simulink model "hyd_hyb_2_int_cont_Final_AMT"  (R2013b)
settings: Solver=ode4  StartTime=0  StopTime=3005  FixedStep=0.01  MaxStep=.4  RelTol=1e-8
InitFcn:
  | const_3_new
values from neighbouring files (symbols this model uses):
  Af = 6.3    [brk_enrg.m]    (also in brk_enrg_1.m)
  BSFC_906_205 = [3.5684 4.3466 5.1668 6.0769 6.988 7.8992 8.8104 9.7336 10.8548 11.9809 13.1112 14.2571 ... (663 elements, 39x17)]    [BSFC_map_906_205.mat]
  Cd = 0.55    [brk_enrg.m]    (also in brk_enrg_1.m)
  den = 1.202    [brk_enrg.m]    (also in brk_enrg_1.m)
  fr = 0.01    [brk_enrg.m]    (also in brk_enrg_1.m)
undefined symbols (not defined in the file or in its folder): clutchRise, down_spd_2, down_spd_3, down_spd_4, down_spd_c, Driving_Cycle, fuel_density, gearshift, I_wheel, Idle_spd_eng_906, M1_hydr, p_v_15, pmax_125, qv_125, Rw, sec_eng_sfc_map, T0, T1, T_max_906, T_min, TC_spd_ratio_max, teta_new_10, torque_convertor, Twait, up_spd_1, up_spd_2, up_spd_3, up_spd_c, v_p_10, v_p_15, v_p_5
libraries: neural x1742, fl_lib x43, nesl_utility x30, sdl_lib x14, simulink x4, simulink_need_slupdate x1
(part 11 of 26)

== system hyd_hyb_2_int_cont_Final_AMT/controller1/optimized controller/SOC upper 0.5/SOC under 0.6/net_col_e_f_5_6/Layer 2/LW{2,1} ==
  "ad{2,1}" : Inport  PortDimensions=30
  "IW{2,1}(1,:)'" : Constant  Value=[-0.030393832532962472;-0.2140586465492049;-0.31177410134924299;-0.46613714335472767;-0.201873752791425;-0.35802654413849078;0.41211751545428793;-0.35557829317260753;0.17263895513984945;-0.21666908912043678;-0.13972381535234679;-0.019824875407318664;0.17842229946428553;0.044381204849071522;-0.32894732465246224;-0.12171008049632184;0.13814590271554272;0.31343496753063571;0.49075574510674602;-0.07753439785263945;-0.11371475039833147;-0.43264143413308215;-0.31682924708133714;0.45184843514620843;-0.10010733916402992;-0.073217200056284279;0.33498722182306373;0.2080296291338882;-0.34019436744511455;-0.12407925676720709]
  "IW{2,1}(10,:)'" : Constant  Value=[-0.2505704282524524;-0.3939257554207935;-0.29975165870681642;-0.15031973290133904;-0.24045771892346329;-0.24216831733474872;0.34991520385977254;0.056483630435657121;0.075039420272193916;0.040783928391016355;-0.17972854864617466;0.37100873007899093;0.3223440043286851;0.083094181567428288;-0.34343211957443465;-0.24139719218091207;-0.23310945944076636;-0.19630209941555543;-0.39839647141125911;-0.086263558874944163;0.084290908148239183;0.46372794004131584;0.30745835414815731;0.4667718683031023;0.38177352303007822;0.39526221301583331;0.037058129894969059;-0.033237412446624953;0.085864544510327004;-0.4416572811793027]
  "IW{2,1}(2,:)'" : Constant  Value=[-0.28762870212077329;0.054589128164715936;0.43070941004987917;-0.19143207832331097;0.0318475712201398;-0.053702387359868146;0.3782037039878825;-0.10929522120960172;0.02340575506249706;0.1208551424159988;-0.32907776200005534;-0.29614820983664508;-0.04883438578651441;0.2945504283388431;0.38772134611455616;-0.1426067233264004;0.34279273527863979;-0.42587520602132178;0.30745629555523329;0.085481158280511255;-0.31301428028501527;0.45433653176700362;-0.34548226823741135;0.45162137833646937;-0.19606462470782865;-0.44727339366708768;-0.32633196267115394;-0.022768106510234126;0.19019249866074842;0.12534221654070224]
  "IW{2,1}(3,:)'" : Constant  Value=[0.39112741680931812;-0.31978339521640231;-0.45618332838328646;0.22187613151776697;0.15902090508890185;0.083633472465386507;0.068775436612897214;-0.27468778024818002;-0.0095156153879017956;-0.3329705145032763;-0.41709465282714198;-0.083926949400729201;-0.43867924463374353;-0.47594030290625516;0.37055116856733306;-0.30038080956129914;-0.19346252510558046;-0.071156466707070598;-0.1565410346606585;0.31532679870256697;-0.25473325292829679;0.33712413893538379;-0.085088376218202588;-0.17938172910409972;0.24970446460562623;-0.33450621725925617;-0.17977936758544141;0.30664510288542302;-0.068953816926079908;-0.13239439222807625]
  "IW{2,1}(4,:)'" : Constant  Value=[0.5236702898730865;0.21199966696477551;0.35952752928707649;0.019723530590060441;0.44209036013212977;-0.045784888845008344;0.54989711619444792;-0.047025448166544644;-0.036356167286904967;0.24149337951075159;-0.36033388484015128;0.15509905661754866;0.24429431465823442;0.56993242132756905;-0.046193773380533189;-0.16184817194805917;0.17925337861437229;0.46969723879260278;0.34350789605630055;0.08863875089456541;0.20464674967063287;0.21542542386226093;-0.30757414976248237;0.22245003609036712;0.099301281549722578;0.04057872191728587;-0.33201719417637826;-0.47694799309855712;-0.33359512873481728;-0.33443453741741941]
  "IW{2,1}(5,:)'" : Constant  Value=[-0.39959821967519593;-0.31362810096707033;-0.31682724713016341;0.39862604414021602;-0.36168966900035454;-0.38588696726317745;-0.15797698948252611;-0.090531432147917826;-0.33017756180156344;-0.36582779220206285;-0.16339659393293465;0.30719233431666931;-0.37016484251633996;0.344361440321791;-0.17456285655515369;0.2131417301444393;-0.32163373894503566;-0.29509333147520467;0.14907288465152124;-0.31687539569313966;0.11409578709933664;0.16969225538936128;-0.1613998950013931;0.11147161080246354;0.11126677588053642;-0.10582537476789625;0.37764324773258484;-0.25725888409799397;0.17346828146213097;0.2968195483551983]
  "IW{2,1}(6,:)'" : Constant  Value=[-0.11716752768262495;0.20377807736649567;0.39051919150098868;-0.10068145034167778;-0.45898166603392643;0.14044780715231203;0.3766843442574494;-0.31621402495343004;0.40628439400051353;0.0026886561759890833;-0.23275447184164255;0.11741623482208553;-0.47709346258154012;0.029795882252597751;0.27610056922766701;0.11975856223889453;-0.23493711394866479;0.39441111981074417;-0.1305257437571978;-0.3096269494893204;0.21423914366738864;0.29007697061490489;-0.37128870036285971;-0.17096385603206457;-0.33949208301054939;-0.20358861932336775;-0.103794175225949;-0.12728191492578217;0.073028592828514385;0.50715491081104047]
  "IW{2,1}(7,:)'" : Constant  Value=[0.22889715197947469;-0.14817850016315076;0.29384797220436742;-0.17292464780674385;0.039905368244081973;0.51560989905964549;-0.019104485775315299;0.00450671459486187;-0.24885944976112842;0.11294055983311714;-0.35984134998870648;0.56660710621235377;0.4502529330165625;-0.12729977158914091;-0.25887898451001889;-0.4202593621623692;0.079298806675420247;0.23489367335784675;-0.36990629226240712;0.049141324657233795;0.16139682719459081;-0.30821522108094518;0.13499998583520637;-0.089586453672634944;0.38220329351721338;-0.26661160481608931;-0.14550662761818581;-0.13187580715835978;-0.11647199599773699;0.26317272202300696]
  "IW{2,1}(8,:)'" : Constant  Value=[0.044685744582128734;-0.1908844366489017;-0.174794908065215;0.32643162068799214;-0.37050611537088302;-0.32225071082540269;-0.29490940136720639;0.05038227814640945;-0.42624323738224995;0.39773459662235627;-0.30823260303902394;0.18941270558875947;0.076728852910635137;-0.24291076735984238;0.040687603382098023;0.38406554522818398;-0.12119441015776648;0.54700185417442515;0.092888736216969123;0.015603285313999743;-0.4911935537467782;-0.024179836928880958;-0.14313432950027993;-0.14638852747492093;0.40459554299034611;-0.37124396054958153;0.4052460971208755;-0.1241390298447143;0.22476477752652688;0.17000260780043774]
  "IW{2,1}(9,:)'" : Constant  Value=[0.40187325571425492;0.25449281632989129;-0.076943631829698544;-0.21240760751343882;0.040048997970771043;0.19620197480948465;-0.37138567337556944;0.39831762613048866;-0.28931266215843032;-0.39729083923611486;-0.46921791995515649;0.51412890115003618;0.31379829123446729;0.095315428974239447;-0.44370143634003684;-0.33140964460964284;-0.27278751479859847;-0.42011098303670114;-0.024084561465198988;0.10358437043932962;0.64313064936086206;-0.081503436078471866;-0.11002880065828506;-0.23916583284587656;0.23096285494640126;-0.19893311012086728;0.28091952945331422;-0.046984031602095543;0.24418233822697555;0.24118329610468914]
  Mux : Mux  Inputs=10
  dotprod{1..10} (10 alike) : neural/Weight Functions/dotprod
  "lz{2,1}" : Outport
  wires:
  "IW{2,1}(1,:)'"/1 -> dotprod1/1
  "ad{2,1}"/1 -> dotprod1/2, dotprod2/2, dotprod3/2, dotprod4/2, dotprod5/2, dotprod6/2, dotprod7/2, dotprod8/2, dotprod9/2, dotprod10/2
  dotprod1/1 -> Mux/1
  "IW{2,1}(2,:)'"/1 -> dotprod2/1
  dotprod2/1 -> Mux/2
  "IW{2,1}(3,:)'"/1 -> dotprod3/1
  dotprod3/1 -> Mux/3
  "IW{2,1}(4,:)'"/1 -> dotprod4/1
  dotprod4/1 -> Mux/4
  "IW{2,1}(5,:)'"/1 -> dotprod5/1
  dotprod5/1 -> Mux/5
  "IW{2,1}(6,:)'"/1 -> dotprod6/1
  dotprod6/1 -> Mux/6
  "IW{2,1}(7,:)'"/1 -> dotprod7/1
  dotprod7/1 -> Mux/7
  "IW{2,1}(8,:)'"/1 -> dotprod8/1
  dotprod8/1 -> Mux/8
  "IW{2,1}(9,:)'"/1 -> dotprod9/1
  dotprod9/1 -> Mux/9
  "IW{2,1}(10,:)'"/1 -> dotprod10/1
  dotprod10/1 -> Mux/10
  Mux/1 -> "lz{2,1}"/1

== system hyd_hyb_2_int_cont_Final_AMT/controller1/optimized controller/SOC upper 0.5/SOC under 0.6/net_col_e_f_5_6/Layer 3/Delays 1 ==
  "p{3}" : Inport  PortDimensions=10
  mux : Mux  Inputs=1
  "pd{3,2}" : Outport
  wires:
  "p{3}"/1 -> mux/1
  mux/1 -> "pd{3,2}"/1

== system hyd_hyb_2_int_cont_Final_AMT/controller1/optimized controller/SOC upper 0.5/SOC under 0.6/net_col_e_f_5_6/Layer 3/LW{3,2} ==
  "ad{3,2}" : Inport  PortDimensions=10
  "IW{3,2}(1,:)'" : Constant  Value=[0.6820311486021321;-0.48687596019537038;-0.099773750784149948;0.92745064423738854;0.58814782146156741;-0.41412122914754468;-0.27711602366879279;0.34179434137314957;-0.92605251129828714;1.0113598211442618]
  Mux : Mux  Inputs=1
  dotprod1 : neural/Weight Functions/dotprod
  "lz{3,2}" : Outport
  wires:
  "IW{3,2}(1,:)'"/1 -> dotprod1/1
  "ad{3,2}"/1 -> dotprod1/2
  dotprod1/1 -> Mux/1
  Mux/1 -> "lz{3,2}"/1

== system hyd_hyb_2_int_cont_Final_AMT/controller1/optimized controller/SOC upper 0.5/SOC under 0.6/net_loc_rod_5_6/Layer 1/Delays 1 ==
  "p{1}" : Inport  PortDimensions=2
  mux : Mux  Inputs=1
  "pd{1,1}" : Outport
  wires:
  "p{1}"/1 -> mux/1
  mux/1 -> "pd{1,1}"/1

== system hyd_hyb_2_int_cont_Final_AMT/controller1/optimized controller/SOC upper 0.5/SOC under 0.6/net_loc_rod_5_6/Layer 1/IW{1,1} ==
  "pd{1,1}" : Inport  PortDimensions=2
  "IW{1,1}(1,:)'" : Constant  Value=[-6.7309330170199999;5.7367344667021127]
  "IW{1,1}(10,:)'" : Constant  Value=[-8.7922870682239527;1.0330077469568615]
  "IW{1,1}(11,:)'" : Constant  Value=[6.9837130293121303;5.4192670047826033]
  "IW{1,1}(12,:)'" : Constant  Value=[4.325460244122568;7.7438798911268565]
  "IW{1,1}(13,:)'" : Constant  Value=[-6.3344127461650013;6.1856486901229077]
  "IW{1,1}(14,:)'" : Constant  Value=[-1.9733514180291731;-8.6238469824021387]
  "IW{1,1}(15,:)'" : Constant  Value=[-2.3605885459119227;-8.5314691020515863]
  "IW{1,1}(16,:)'" : Constant  Value=[-4.8892080793798369;7.3866903131456692]
  "IW{1,1}(17,:)'" : Constant  Value=[5.8569397262097889;6.7096509511682889]
  "IW{1,1}(18,:)'" : Constant  Value=[-4.4027205889575827;7.6822038939167063]
  "IW{1,1}(19,:)'" : Constant  Value=[8.7792518860140909;1.1591702425203565]
  "IW{1,1}(2,:)'" : Constant  Value=[6.2678488323062229;6.251648838835326]
  "IW{1,1}(20,:)'" : Constant  Value=[-7.9610155557707865;-3.8802632991194277]
  "IW{1,1}(21,:)'" : Constant  Value=[5.755058346987636;6.7197585570713629]
  "IW{1,1}(22,:)'" : Constant  Value=[7.3858749888249431;-4.8854449488948442]
  "IW{1,1}(23,:)'" : Constant  Value=[-2.5028469102563147;-8.4893261832660354]
  "IW{1,1}(24,:)'" : Constant  Value=[8.50910667173771;-2.4597062713706324]
  "IW{1,1}(25,:)'" : Constant  Value=[-8.2476309100150864;3.2111046237292071]
  "IW{1,1}(26,:)'" : Constant  Value=[-4.0253091511868995;-7.862701807156669]
  "IW{1,1}(27,:)'" : Constant  Value=[2.2947605364640964;8.551294247952935]
  "IW{1,1}(28,:)'" : Constant  Value=[0.90305404500173392;-8.8024864439756705]
  "IW{1,1}(29,:)'" : Constant  Value=[7.0857227926174824;-5.297360563446083]
  "IW{1,1}(3,:)'" : Constant  Value=[8.4767942670534939;2.5639295625443186]
  "IW{1,1}(30,:)'" : Constant  Value=[-5.6140927717680311;-6.8589023719873676]
  "IW{1,1}(31,:)'" : Constant  Value=[-5.8556189515114712;6.6477437525997107]
  "IW{1,1}(32,:)'" : Constant  Value=[1.520259467845865;8.7265416088585415]
  "IW{1,1}(33,:)'" : Constant  Value=[-7.4255785682577606;-4.8121870145571606]
  "IW{1,1}(34,:)'" : Constant  Value=[3.7334199192712054;-7.9252934165752285]
  "IW{1,1}(35,:)'" : Constant  Value=[-8.8434135803568381;0.098556138484456934]
  "IW{1,1}(36,:)'" : Constant  Value=[8.7558988672878311;-1.1835294834309311]
  "IW{1,1}(37,:)'" : Constant  Value=[-6.3607928740217332;6.2831314432408085]
  "IW{1,1}(38,:)'" : Constant  Value=[-2.1369631047449062;-8.5869236354604546]
  "IW{1,1}(39,:)'" : Constant  Value=[-3.7481499623866923;8.0515766767633732]
  "IW{1,1}(4,:)'" : Constant  Value=[5.9639192573581292;-6.5449514183387238]
  "IW{1,1}(40,:)'" : Constant  Value=[-8.8210912896683222;1.1388181613834201]
  "IW{1,1}(5,:)'" : Constant  Value=[6.0684708526836246;6.4470542210774306]
  "IW{1,1}(6,:)'" : Constant  Value=[0.14739906835272285;8.8139730930743863]
  "IW{1,1}(7,:)'" : Constant  Value=[-4.8674516940697989;7.4037526818854085]
  "IW{1,1}(8,:)'" : Constant  Value=[5.18948242438666;-7.1849747561483799]
  "IW{1,1}(9,:)'" : Constant  Value=[-6.3190502504535511;-6.2049133477751708]
  Mux : Mux  Inputs=40
  dotprod{1..40} (40 alike) : neural/Weight Functions/dotprod
  "iz{1,1}" : Outport
  wires:
  "IW{1,1}(1,:)'"/1 -> dotprod1/1
  "pd{1,1}"/1 -> dotprod1/2, dotprod2/2, dotprod3/2, dotprod4/2, dotprod5/2, dotprod6/2, dotprod7/2, dotprod8/2, dotprod9/2, dotprod10/2, dotprod11/2, dotprod12/2, dotprod13/2, dotprod14/2, dotprod15/2, dotprod16/2, dotprod17/2, dotprod18/2, dotprod19/2, dotprod20/2, dotprod21/2, dotprod22/2, dotprod23/2, dotprod24/2, dotprod25/2, dotprod26/2, dotprod27/2, dotprod28/2, dotprod29/2, dotprod30/2, dotprod31/2, dotprod32/2, dotprod33/2, dotprod34/2, dotprod35/2, dotprod36/2, dotprod37/2, dotprod38/2, dotprod39/2, dotprod40/2
  dotprod1/1 -> Mux/1
  "IW{1,1}(2,:)'"/1 -> dotprod2/1
  dotprod2/1 -> Mux/2
  "IW{1,1}(3,:)'"/1 -> dotprod3/1
  dotprod3/1 -> Mux/3
  "IW{1,1}(4,:)'"/1 -> dotprod4/1
  dotprod4/1 -> Mux/4
  "IW{1,1}(5,:)'"/1 -> dotprod5/1
  dotprod5/1 -> Mux/5
  "IW{1,1}(6,:)'"/1 -> dotprod6/1
  dotprod6/1 -> Mux/6
  "IW{1,1}(7,:)'"/1 -> dotprod7/1
  dotprod7/1 -> Mux/7
  "IW{1,1}(8,:)'"/1 -> dotprod8/1
  dotprod8/1 -> Mux/8
  "IW{1,1}(9,:)'"/1 -> dotprod9/1
  dotprod9/1 -> Mux/9
  "IW{1,1}(10,:)'"/1 -> dotprod10/1
  dotprod10/1 -> Mux/10
  "IW{1,1}(11,:)'"/1 -> dotprod11/1
  dotprod11/1 -> Mux/11
  "IW{1,1}(12,:)'"/1 -> dotprod12/1
  dotprod12/1 -> Mux/12
  "IW{1,1}(13,:)'"/1 -> dotprod13/1
  dotprod13/1 -> Mux/13
  "IW{1,1}(14,:)'"/1 -> dotprod14/1
  dotprod14/1 -> Mux/14
  "IW{1,1}(15,:)'"/1 -> dotprod15/1
  dotprod15/1 -> Mux/15
  "IW{1,1}(16,:)'"/1 -> dotprod16/1
  dotprod16/1 -> Mux/16
  "IW{1,1}(17,:)'"/1 -> dotprod17/1
  dotprod17/1 -> Mux/17
  "IW{1,1}(18,:)'"/1 -> dotprod18/1
  dotprod18/1 -> Mux/18
  "IW{1,1}(19,:)'"/1 -> dotprod19/1
  dotprod19/1 -> Mux/19
  "IW{1,1}(20,:)'"/1 -> dotprod20/1
  dotprod20/1 -> Mux/20
  "IW{1,1}(21,:)'"/1 -> dotprod21/1
  dotprod21/1 -> Mux/21
  "IW{1,1}(22,:)'"/1 -> dotprod22/1
  dotprod22/1 -> Mux/22
  "IW{1,1}(23,:)'"/1 -> dotprod23/1
  dotprod23/1 -> Mux/23
  "IW{1,1}(24,:)'"/1 -> dotprod24/1
  dotprod24/1 -> Mux/24
  "IW{1,1}(25,:)'"/1 -> dotprod25/1
  dotprod25/1 -> Mux/25
  "IW{1,1}(26,:)'"/1 -> dotprod26/1
  dotprod26/1 -> Mux/26
  "IW{1,1}(27,:)'"/1 -> dotprod27/1
  dotprod27/1 -> Mux/27
  "IW{1,1}(28,:)'"/1 -> dotprod28/1
  dotprod28/1 -> Mux/28
  "IW{1,1}(29,:)'"/1 -> dotprod29/1
  dotprod29/1 -> Mux/29
  "IW{1,1}(30,:)'"/1 -> dotprod30/1
  dotprod30/1 -> Mux/30
  "IW{1,1}(31,:)'"/1 -> dotprod31/1
  dotprod31/1 -> Mux/31
  "IW{1,1}(32,:)'"/1 -> dotprod32/1
  dotprod32/1 -> Mux/32
  "IW{1,1}(33,:)'"/1 -> dotprod33/1
  dotprod33/1 -> Mux/33
  "IW{1,1}(34,:)'"/1 -> dotprod34/1
  dotprod34/1 -> Mux/34
  "IW{1,1}(35,:)'"/1 -> dotprod35/1
  dotprod35/1 -> Mux/35
  "IW{1,1}(36,:)'"/1 -> dotprod36/1
  dotprod36/1 -> Mux/36
  "IW{1,1}(37,:)'"/1 -> dotprod37/1
  dotprod37/1 -> Mux/37
  "IW{1,1}(38,:)'"/1 -> dotprod38/1
  dotprod38/1 -> Mux/38
  "IW{1,1}(39,:)'"/1 -> dotprod39/1
  dotprod39/1 -> Mux/39
  "IW{1,1}(40,:)'"/1 -> dotprod40/1
  dotprod40/1 -> Mux/40
  Mux/1 -> "iz{1,1}"/1

== system hyd_hyb_2_int_cont_Final_AMT/controller1/optimized controller/SOC upper 0.5/SOC under 0.6/net_loc_rod_5_6/Layer 2/Delays 1 ==
  "p{2}" : Inport  PortDimensions=40
  mux : Mux  Inputs=1
  "pd{2,1}" : Outport
  wires:
  "p{2}"/1 -> mux/1
  mux/1 -> "pd{2,1}"/1
